simulink model "gm_sampleModel1894_4_sub"  (R2023a)
settings: Solver=VariableStepAuto  StartTime=0.0  StopTime=10.0  RelTol=1e-3
libraries: simulink x3
settings Model: Creator=user1  LastModifiedBy=user1
settings OptimizationCC: BlockReduction=off  ConditionallyExecuteInputs=off
settings DebuggingCC: InheritedTsInSrcMsg=none

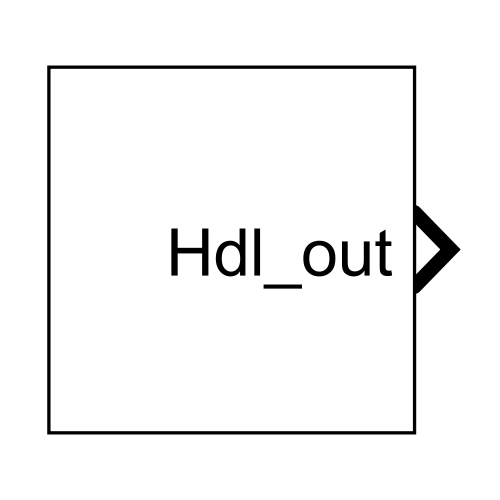
[thumbnail: Simulink's stored preview of the top-level diagram]
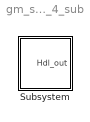
== system gm_sampleModel1894_4_sub ==
  Subsystem : Subsystem

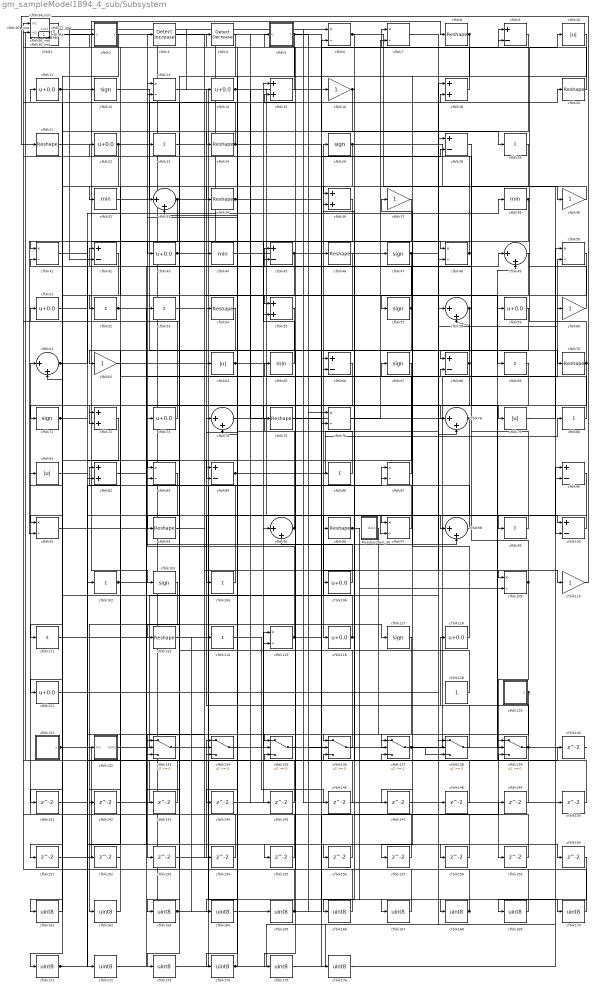
== system gm_sampleModel1894_4_sub/Subsystem ==
  Mysubsystem_30 : Subsystem
  cfblk1 : simulink/Logic and Bit Operations/Detect Increase  vinit=0.0  OutDataTypeStr=uint8
      settings: LibrarySourceBlock=|
      | hdlsllib/Logic and Bit
      | Operations/Detect
      | Increase
  cfblk{10,64,79,81} (4 alike) : Abs  OutDataTypeStr=uint8  SaturateOnIntegerOverflow=off
  cfblk{9,28,42,45,66,68,84,90,100} (9 alike) : Sum  Inputs=+-  OutDataTypeStr=uint8
  cfblk101_inst : Subsystem
  cfblk{23,29,52..53,69,80,86,99,102,104,111,114} (12 alike) : Sum  Inputs=+  OutDataTypeStr=uint8
  cfblk{12,26,47,57,67,71,103,117} (8 alike) : Signum
  cfblk{11,14,22,43,51,59,73,106,116,118,121} (11 alike) : Bias  Bias=0.0  SaturateOnIntegerOverflow=off
  cfblk{6..7,13,41,48,50,76,83,87,91,97,109,115} (13 alike) : Product  Inputs=*/  OutDataTypeStr=uint8  RndMeth=Zero  SaturateOnIntegerOverflow=on
  cfblk{16,37,40,60,62,110} (6 alike) : Gain  OutDataTypeStr=uint8
  cfblk{8,20..21,24,34,46,54,70,75,93,96,113} (12 alike) : Reshape
  cfblk120_inst : Subsystem
  cfblk128 : Constant  OutDataTypeStr=uint8  SampleTime=-1
  cfblk129 : Subsystem  mask(Counter Free-Running){NumBits=double(16), tsamp=double(-1)}
      mask prompts: NumBits "Simulink:masks:NumberOfBits_MP"; tsamp "Simulink:masks:SampleTime_MP"
      mask help: Simulink:masks:CounterFreeRunning_MD
  cfblk131 : Subsystem  mask(Counter Limited){uplimit=double(7), tsamp=double(-1)}
      mask prompts: uplimit "Simulink:masks:UpperLimit_MP"; tsamp "Simulink:masks:SampleTime_MP"
      mask help: Simulink:masks:CounterLimited_MD
      mask init:
      | nbits = double(8);
      | tsamp = double(-1);
      | uplimit = double(7);
  cfblk132 : Subsystem
  cfblk{133..139} (7 alike) : Switch  OutDataTypeStr=uint8  SaturateOnIntegerOverflow=off  InputSameDT=off
  cfblk{140..160} (21 alike) : Delay  SampleTime=1
  cfblk{15,18,36,55,72,82} (6 alike) : Sum  OutDataTypeStr=uint8
  cfblk{161..176} (16 alike) : DataTypeConversion  OutDataTypeStr=uint8  SaturateOnIntegerOverflow=off  RndMeth=Floor
  cfblk2 : Subsystem  mask(Compare To Constant){relop=<=, const=double(3), OutDataTypeStr=uint8, ZeroCross=on}
      mask prompts: relop "Simulink:masks:Operator_MP"; const "Simulink:masks:ConstantValue_MP"; OutDataTypeStr "Simulink:masks:OutputDataType_MP"; ZeroCross "Simulink:masks:EnableZerocrossingDetection_MP"
      mask help: Simulink:masks:CompareToConstant_MD
      mask init:
      | OutDataTypeStr = 'uint8';
      | ZeroCross = 'on';
      | blkName = 'sampleModel1894_4_sub/Subsystem/cfblk2';
      | const = double(3);
      | const_str = '3.0';
      | const_val = double(3);
      | relop = '<=';
      | setValue = 'fixdt(0, 8)';
      | str = '<= 3';
      mask TypeOptions relop: == | ~= | < | <= | >= | >
      mask TypeOptions OutDataTypeStr: Simulink:masks:uint8 | Simulink:masks:boolean
      mask Callback ZeroCross: sl('zeroCrossEnable', gcbh);
      mask Display: disp(str)
  cfblk3 : simulink/Logic and Bit Operations/Detect Increase  vinit=0.0  OutDataTypeStr=uint8
      settings: LibrarySourceBlock=|
      | hdlsllib/Logic and Bit
      | Operations/Detect
      | Increase
  cfblk30_inst : Subsystem
  cfblk{32,39,44,65} (4 alike) : MinMax  OutDataTypeStr=uint8
  cfblk{33,49,58,61,74,78,95,98} (8 alike) : Sum  Inputs=|++  OutDataTypeStr=uint8
  cfblk4 : simulink/Logic and Bit Operations/Detect Decrease  vinit=0.0  OutDataTypeStr=uint8
      settings: LibrarySourceBlock=|
      | hdlsllib/Logic and Bit
      | Operations/Detect
      | Decrease
  cfblk5 : Subsystem  mask(Detect Fall Negative){vinit=double(0), InputProcessing=Elements as channels (sample based), OutDataTypeStr=uint8}
      mask prompts: vinit "Simulink:masks:InitialCondition_MP"; InputProcessing "Simulink:masks:InputProcessing_MP"; OutDataTypeStr "Simulink:masks:OutputDataType_MP"
      mask help: Simulink:masks:DetectFallNegative_MD
      mask init:
      | InputProcessing = 'Elements as channels (sample based)';
      | OutDataTypeStr = 'uint8';
      | vinit = double(0);
      mask TypeOptions InputProcessing: Simulink:masks:ColumnsAsChannelsFrameBased | Simulink:masks:ElementsAsChannelsSampleBased
      mask TypeOptions OutDataTypeStr: Simulink:masks:uint8 | Simulink:masks:boolean
      mask Display: fprintf('U < 0\n&  NOT\nU/z < 0')
  cfblk56_inst : Subsystem
  cfblk77_inst : Subsystem
  cfblk94_inst : Subsystem
  Hdl_out : Outport  OutDataTypeStr=uint8  SampleTime=1
  wires:
  Mysubsystem_30/1(Out1) -> cfblk135/1
  cfblk1/1 -> cfblk8/1, cfblk103/1
  cfblk10/1 -> cfblk173/1
  cfblk100/1 -> cfblk116/1
  cfblk101_inst/1(out1) -> cfblk94_inst/1(in1)
  cfblk102/1 -> cfblk98/2, cfblk156/1
  cfblk103/1 -> cfblk162/1
  cfblk104/1 -> cfblk3/1
  cfblk106/1 -> cfblk95/2
  cfblk109/1 -> cfblk41/2, cfblk159/1
  cfblk11/1 -> cfblk97/1, cfblk48/1, cfblk151/1
  cfblk110/1 -> cfblk21/1
  cfblk111/1 -> cfblk26/1
  cfblk113/1 -> cfblk155/1
  cfblk114/1 -> cfblk146/1
  cfblk115/1 -> cfblk73/1, cfblk10/1
  cfblk116/1 -> cfblk166/1, cfblk11/1
  cfblk117/1 -> cfblk153/1
  cfblk118/1 -> cfblk37/1
  cfblk12/1 -> cfblk68/1
  cfblk120_inst/1(out1) -> cfblk165/1
  cfblk121/1 -> cfblk18/1
  cfblk128/1 -> cfblk53/1
  cfblk129/1(y) -> cfblk137/2, cfblk133/3
  cfblk13/1 -> cfblk168/1
  cfblk131/1(y) -> cfblk139/3, cfblk132/1(In1)
  cfblk132/1(Out1) -> cfblk48/2
  cfblk133/1 -> cfblk87/1
  cfblk134/1 -> cfblk115/2
  cfblk135/1 -> cfblk46/1
  cfblk136/1 -> cfblk14/1
  cfblk137/1 -> cfblk138/3, cfblk50/2
  cfblk138/1 -> cfblk118/1
  cfblk139/1 -> cfblk54/1, cfblk136/3
  cfblk14/1 -> cfblk100/1, cfblk145/1
  cfblk140/1 -> cfblk1/1
  cfblk141/1 -> cfblk172/1
  cfblk142/1 -> cfblk138/1
  cfblk143/1 -> cfblk30_inst/2(in2)
  cfblk144/1 -> cfblk139/1
  cfblk145/1 -> cfblk115/1
  cfblk146/1 -> cfblk101_inst/2(in2)
  cfblk147/1 -> cfblk78/2
  cfblk148/1 -> cfblk36/2
  cfblk149/1 -> cfblk138/2
  cfblk15/1 -> cfblk30_inst/1(in1)
  cfblk150/1 -> cfblk77_inst/2(in2)
  cfblk151/1 -> cfblk6/2
  cfblk152/1 -> cfblk82/1
  cfblk153/1 -> cfblk134/1
  cfblk154/1 -> cfblk42/1
  cfblk155/1 -> cfblk61/1
  cfblk156/1 -> cfblk15/2
  cfblk157/1 -> cfblk134/3
  cfblk158/1 -> cfblk94_inst/2(in2)
  cfblk159/1 -> cfblk45/1
  cfblk16/1 -> cfblk24/1, cfblk106/1
  cfblk160/1 -> cfblk169/1
  cfblk161/1 -> cfblk81/1
  cfblk162/1 -> cfblk2/1(u)
  cfblk163/1 -> cfblk59/1, cfblk114/1
  cfblk164/1 -> cfblk4/1
  cfblk165/1 -> cfblk51/1, cfblk76/1, cfblk149/1
  cfblk166/1 -> cfblk120_inst/1(in1)
  cfblk167/1 -> cfblk120_inst/2(in2)
  cfblk168/1 -> cfblk75/1, cfblk135/3
  cfblk169/1 -> cfblk13/1
  cfblk170/1 -> cfblk13/2
  cfblk171/1 -> cfblk137/3, cfblk87/2, cfblk140/1
  cfblk172/1 -> cfblk49/1
  cfblk173/1 -> cfblk49/2
  cfblk174/1 -> cfblk74/1, cfblk148/1
  cfblk175/1 -> cfblk90/1
  cfblk176/1 -> cfblk90/2
  cfblk18/1 -> cfblk77_inst/1(in1)
  cfblk2/1(y) -> cfblk161/1
  cfblk20/1 -> cfblk9/1
  cfblk21/1 -> cfblk55/2
  cfblk22/1 -> cfblk18/2, cfblk121/1
  cfblk23/1 -> cfblk109/1
  cfblk24/1 -> cfblk66/1, cfblk101_inst/1(in1)
  cfblk26/1 -> cfblk93/1, cfblk113/1, cfblk40/1, cfblk52/1
  cfblk28/1 -> cfblk78/1
  cfblk29/1 -> cfblk133/1
  cfblk3/1 -> cfblk55/1
  cfblk30_inst/1(out1) -> cfblk6/1
  cfblk32/1 -> cfblk20/1
  cfblk33/1 -> cfblk136/2, cfblk91/1
  cfblk34/1 -> cfblk176/1, cfblk167/1
  cfblk36/1 -> cfblk43/1
  cfblk37/1 -> cfblk82/2
  cfblk39/1 -> cfblk91/2, cfblk157/1
  cfblk4/1 -> cfblk163/1
  cfblk40/1 -> cfblk32/1
  cfblk41/1 -> cfblk102/1
  cfblk42/1 -> cfblk61/2
  cfblk43/1 -> cfblk45/2, cfblk69/1
  cfblk44/1 -> cfblk96/1
  cfblk45/1 -> cfblk71/1, cfblk28/2
  cfblk46/1 -> cfblk62/1
  cfblk47/1 -> cfblk136/1, cfblk110/1
  cfblk48/1 -> cfblk56_inst/2(in2), cfblk28/1
  cfblk49/1 -> cfblk171/1
  cfblk5/1(Y) -> cfblk74/2, cfblk34/1, cfblk29/1
  cfblk50/1 -> cfblk147/1
  cfblk51/1 -> cfblk98/1
  cfblk52/1 -> cfblk117/1, cfblk76/2
  cfblk53/1 -> cfblk70/1
  cfblk54/1 -> cfblk83/1
  cfblk55/1 -> cfblk164/1
  cfblk56_inst/1(out1) -> cfblk150/1
  cfblk57/1 -> cfblk72/2, cfblk137/1, cfblk44/1
  cfblk58/1 -> cfblk143/1, cfblk142/1
  cfblk59/1 -> cfblk175/1
  cfblk6/1 -> cfblk36/1, cfblk100/2
  cfblk60/1 -> cfblk7/1
  cfblk61/1 -> cfblk158/1, cfblk39/1
  cfblk62/1 -> cfblk95/1
  cfblk64/1 -> cfblk68/2, cfblk139/2
  cfblk65/1 -> cfblk15/1
  cfblk66/1 -> cfblk72/1
  cfblk67/1 -> cfblk144/1
  cfblk68/1 -> cfblk66/2, cfblk58/2, cfblk152/1
  cfblk69/1 -> cfblk141/1
  cfblk7/1 -> cfblk58/1
  cfblk70/1 -> cfblk9/2, cfblk135/2
  cfblk71/1 -> cfblk84/2, cfblk99/1
  cfblk72/1 -> cfblk111/1
  cfblk73/1 -> cfblk56_inst/1(in1)
  cfblk74/1 -> cfblk79/1
  cfblk75/1 -> cfblk160/1
  cfblk76/1 -> cfblk7/2
  cfblk77_inst/1(out1) -> cfblk47/1, cfblk16/1
  cfblk78/1 -> cfblk97/2, Hdl_out/1, cfblk104/1
  cfblk79/1 -> cfblk50/1
  cfblk8/1 -> cfblk84/1, cfblk57/1
  cfblk80/1 -> cfblk22/1
  cfblk81/1 -> cfblk134/2
  cfblk82/1 -> cfblk65/1
  cfblk83/1 -> cfblk133/2
  cfblk84/1 -> cfblk60/1, cfblk80/1
  cfblk86/1 -> cfblk5/1(U)
  cfblk87/1 -> cfblk67/1
  cfblk9/1 -> cfblk41/1
  cfblk90/1 -> cfblk174/1
  cfblk91/1 -> cfblk64/1
  cfblk93/1 -> cfblk154/1
  cfblk94_inst/1(out1) -> cfblk42/2, cfblk12/1
  cfblk95/1 -> cfblk33/2, cfblk33/1
  cfblk96/1 -> cfblk170/1, cfblk109/2
  cfblk97/1 -> cfblk86/1
  cfblk98/1 -> cfblk83/2
  cfblk99/1 -> cfblk23/1

== system gm_sampleModel1894_4_sub/Subsystem/Mysubsystem_30 ==
  cfblk130 : Subsystem  mask(Counter Free-Running){NumBits=double(16), tsamp=double(-1)}
      mask prompts: NumBits "Simulink:masks:NumberOfBits_MP"; tsamp "Simulink:masks:SampleTime_MP"
      mask help: Simulink:masks:CounterFreeRunning_MD
  cfblk63 : MinMax
  Out1 : Outport  SampleTime=1
  wires:
  cfblk130/1(y) -> cfblk63/1
  cfblk63/1 -> Out1/1

== system gm_sampleModel1894_4_sub/Subsystem/cfblk101_inst ==
  in1 : Inport  OutDataTypeStr=uint8  SampleTime=1
  in2 : Inport  Port=2  OutDataTypeStr=uint8  SampleTime=1
  mul_cfblk101_dotp_mulcomp : Product  Inputs=**  OutDataTypeStr=uint8  SampleTime=1
  out1 : Outport  OutDataTypeStr=uint8  SampleTime=1
  wires:
  in1/1 -> mul_cfblk101_dotp_mulcomp/1
  in2/1 -> mul_cfblk101_dotp_mulcomp/2
  mul_cfblk101_dotp_mulcomp/1 -> out1/1

== system gm_sampleModel1894_4_sub/Subsystem/cfblk120_inst ==
  in1 : Inport  OutDataTypeStr=uint8  SampleTime=1
  in2 : Inport  Port=2  OutDataTypeStr=uint8  SampleTime=1
  mul_cfblk120_dotp_mulcomp : Product  Inputs=**  OutDataTypeStr=uint8  SampleTime=1
  out1 : Outport  OutDataTypeStr=uint8  SampleTime=1
  wires:
  in1/1 -> mul_cfblk120_dotp_mulcomp/1
  in2/1 -> mul_cfblk120_dotp_mulcomp/2
  mul_cfblk120_dotp_mulcomp/1 -> out1/1

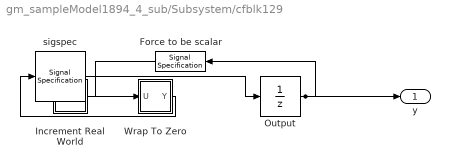
== system gm_sampleModel1894_4_sub/Subsystem/cfblk129 ==
  Force to be scalar : SignalSpecification  DisableCoverage=on  Dimensions=1
  Increment Real World : Subsystem  mask(Real World Value Increment){}
      mask help: Simulink:masks:RealWorldValueIncrement_MD
      mask Display: disp('V++')
  Output : UnitDelay  InitialCondition=0.0  SampleTime=tsamp  HasFrameUpgradeWarning=on
  Wrap To Zero : Subsystem  mask(Wrap To Zero){Threshold=double(65535)}
      mask prompts: Threshold "Simulink:masks:Threshold_MP"
      mask help: Simulink:masks:WrapToZero_MD
  sigspec : SignalSpecification  OutDataTypeStr=uint16  Dimensions=1
  y : Outport  SampleTime=1
  wires:
  Force to be scalar/1 -> Increment Real World/1(u)
  Increment Real World/1(y) -> Wrap To Zero/1(U)
  Output/1 -> Force to be scalar/1, y/1
  Wrap To Zero/1(Y) -> sigspec/1
  sigspec/1 -> Output/1

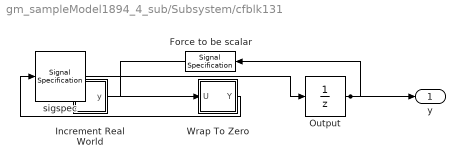
== system gm_sampleModel1894_4_sub/Subsystem/cfblk131 ==
  Force to be scalar : SignalSpecification  DisableCoverage=on  Dimensions=1
  Increment Real World : Subsystem  mask(Real World Value Increment){}
      mask help: Simulink:masks:RealWorldValueIncrement_MD
      mask Display: disp('V++')
  Output : UnitDelay  InitialCondition=0.0  SampleTime=tsamp  HasFrameUpgradeWarning=on
  Wrap To Zero : Subsystem  mask(Wrap To Zero){Threshold=double(7)}
      mask prompts: Threshold "Simulink:masks:Threshold_MP"
      mask help: Simulink:masks:WrapToZero_MD
  sigspec : SignalSpecification  OutDataTypeStr=uint8  Dimensions=1
  y : Outport  SampleTime=1
  wires:
  Force to be scalar/1 -> Increment Real World/1(u)
  Increment Real World/1(y) -> Wrap To Zero/1(U)
  Output/1 -> Force to be scalar/1, y/1
  Wrap To Zero/1(Y) -> sigspec/1
  sigspec/1 -> Output/1

== system gm_sampleModel1894_4_sub/Subsystem/cfblk132 ==
  In1 : Inport  OutDataTypeStr=uint8  PortDimensions=1  SampleTime=1
  Out1 : Outport  SampleTime=1
  wires:
  In1/1 -> Out1/1

== system gm_sampleModel1894_4_sub/Subsystem/cfblk2 ==
  u : Inport  OutDataTypeStr=uint8  SampleTime=1
  Compare : RelationalOperator  Operator=<=  OutDataTypeStr=fixdt(0, 8)
  Constant : Constant  DisableCoverage=on  Value=const  OutDataTypeStr=Inherit: Inherit via back propagation  SampleTime=-1
  y : Outport  SampleTime=1
  wires:
  u/1 -> Compare/1
  Compare/1 -> y/1
  Constant/1 -> Compare/2

== system gm_sampleModel1894_4_sub/Subsystem/cfblk30_inst ==
  in1 : Inport  OutDataTypeStr=uint8  SampleTime=1
  in2 : Inport  Port=2  OutDataTypeStr=uint8  SampleTime=1
  mul_cfblk30_dotp_mulcomp : Product  Inputs=**  OutDataTypeStr=uint8  SampleTime=1
  out1 : Outport  OutDataTypeStr=uint8  SampleTime=1
  wires:
  in1/1 -> mul_cfblk30_dotp_mulcomp/1
  in2/1 -> mul_cfblk30_dotp_mulcomp/2
  mul_cfblk30_dotp_mulcomp/1 -> out1/1

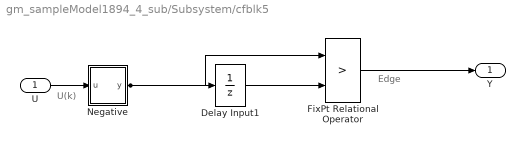
== system gm_sampleModel1894_4_sub/Subsystem/cfblk5 ==
  note: U(k)
  note: Edge
  U : Inport  OutDataTypeStr=uint8  SampleTime=1
  Delay Input1 : UnitDelay  Description=Store in Global RAM  DisableCoverage=on  InitialCondition=vinit  SampleTime=-1  HasFrameUpgradeWarning=on
  FixPt Relational Operator : RelationalOperator  Operator=>  OutDataTypeStr=fixdt(0, 8)  ZeroCross=off  InputSameDT=off
  Negative : Subsystem  mask(Compare To Zero){relop=<, OutDataTypeStr=boolean, ZeroCross=off}
      mask prompts: relop "Simulink:masks:Operator_MP"; OutDataTypeStr "Simulink:masks:OutputDataType_MP"; ZeroCross "Simulink:masks:EnableZerocrossingDetection_MP"
      mask help: Simulink:masks:CompareToZero_MD
      mask init:
      | OutDataTypeStr = 'boolean';
      | ZeroCross = 'off';
      | blkName = 'sampleModel1894_4_sub/Subsystem/cfblk5/Negative';
      | relop = '<';
      | setValue = 'boolean';
      mask TypeOptions relop: == | ~= | < | <= | >= | >
      mask TypeOptions OutDataTypeStr: Simulink:masks:uint8 | Simulink:masks:boolean
      mask Callback ZeroCross: sl('zeroCrossEnable', gcbh);
      mask Display: disp([relop,' 0'])
  Y : Outport  SampleTime=1
  wires:
  U/1 -> Negative/1(u)
  Delay Input1/1 -> FixPt Relational Operator/2
  FixPt Relational Operator/1 -> Y/1
  Negative/1(y) -> FixPt Relational Operator/1, Delay Input1/1

== system gm_sampleModel1894_4_sub/Subsystem/cfblk56_inst ==
  in1 : Inport  OutDataTypeStr=uint8  SampleTime=1
  in2 : Inport  Port=2  OutDataTypeStr=uint8  SampleTime=1
  mul_cfblk56_dotp_mulcomp : Product  Inputs=**  OutDataTypeStr=uint8  SampleTime=1
  out1 : Outport  OutDataTypeStr=uint8  SampleTime=1
  wires:
  in1/1 -> mul_cfblk56_dotp_mulcomp/1
  in2/1 -> mul_cfblk56_dotp_mulcomp/2
  mul_cfblk56_dotp_mulcomp/1 -> out1/1

== system gm_sampleModel1894_4_sub/Subsystem/cfblk77_inst ==
  in1 : Inport  OutDataTypeStr=uint8  SampleTime=1
  in2 : Inport  Port=2  OutDataTypeStr=uint8  SampleTime=1
  mul_cfblk77_dotp_mulcomp : Product  Inputs=**  OutDataTypeStr=uint8  SampleTime=1
  out1 : Outport  OutDataTypeStr=uint8  SampleTime=1
  wires:
  in1/1 -> mul_cfblk77_dotp_mulcomp/1
  in2/1 -> mul_cfblk77_dotp_mulcomp/2
  mul_cfblk77_dotp_mulcomp/1 -> out1/1

== system gm_sampleModel1894_4_sub/Subsystem/cfblk94_inst ==
  in1 : Inport  OutDataTypeStr=uint8  SampleTime=1
  in2 : Inport  Port=2  OutDataTypeStr=uint8  SampleTime=1
  mul_cfblk94_dotp_mulcomp : Product  Inputs=**  OutDataTypeStr=uint8  SampleTime=1
  out1 : Outport  OutDataTypeStr=uint8  SampleTime=1
  wires:
  in1/1 -> mul_cfblk94_dotp_mulcomp/1
  in2/1 -> mul_cfblk94_dotp_mulcomp/2
  mul_cfblk94_dotp_mulcomp/1 -> out1/1

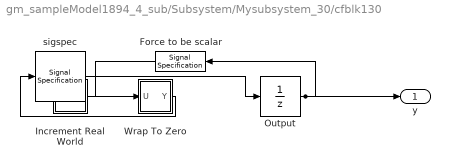
== system gm_sampleModel1894_4_sub/Subsystem/Mysubsystem_30/cfblk130 ==
  Force to be scalar : SignalSpecification  DisableCoverage=on  Dimensions=1
  Increment Real World : Subsystem  mask(Real World Value Increment){}
      mask help: Simulink:masks:RealWorldValueIncrement_MD
      mask Display: disp('V++')
  Output : UnitDelay  InitialCondition=0.0  SampleTime=tsamp  HasFrameUpgradeWarning=on
  Wrap To Zero : Subsystem  mask(Wrap To Zero){Threshold=double(65535)}
      mask prompts: Threshold "Simulink:masks:Threshold_MP"
      mask help: Simulink:masks:WrapToZero_MD
  sigspec : SignalSpecification  OutDataTypeStr=uint16  Dimensions=1
  y : Outport  SampleTime=1
  wires:
  Force to be scalar/1 -> Increment Real World/1(u)
  Increment Real World/1(y) -> Wrap To Zero/1(U)
  Output/1 -> Force to be scalar/1, y/1
  Wrap To Zero/1(Y) -> sigspec/1
  sigspec/1 -> Output/1

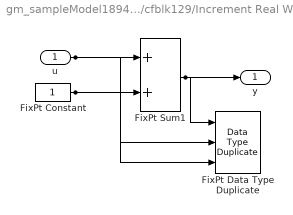
== system gm_sampleModel1894_4_sub/Subsystem/cfblk129/Increment Real World ==
  u : Inport  OutDataTypeStr=uint16  SampleTime=1
  FixPt Constant : Constant  DisableCoverage=on  OutDataTypeStr=Inherit: Inherit via back propagation  SampleTime=-1
  FixPt Data Type Duplicate : DataTypeDuplicate  DisableCoverage=on  NumInputPorts=3
  FixPt Sum1 : Sum  InputSameDT=on  OutDataTypeStr=Inherit: Inherit via back propagation  LockScale=on
  y : Outport  SampleTime=1
  wires:
  u/1 -> FixPt Sum1/1, FixPt Data Type Duplicate/2
  FixPt Constant/1 -> FixPt Sum1/2, FixPt Data Type Duplicate/3
  FixPt Sum1/1 -> FixPt Data Type Duplicate/1, y/1

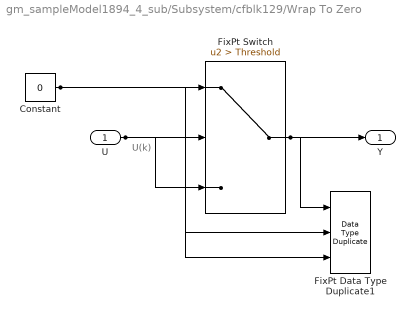
== system gm_sampleModel1894_4_sub/Subsystem/cfblk129/Wrap To Zero ==
  note: U(k)
  U : Inport  OutDataTypeStr=uint16  SampleTime=1
  Constant : Constant  DisableCoverage=on  Value=0  OutDataTypeStr=Inherit: Inherit via back propagation  SampleTime=-1
  FixPt Data Type Duplicate1 : DataTypeDuplicate  DisableCoverage=on  NumInputPorts=3
  FixPt Switch : Switch  Criteria=u2 > Threshold  Threshold=Threshold  OutDataTypeStr=Inherit: Inherit via back propagation  ZeroCross=off  SaturateOnIntegerOverflow=off  InputSameDT=off
  Y : Outport  SampleTime=1
  wires:
  U/1 -> FixPt Switch/3, FixPt Switch/2, FixPt Data Type Duplicate1/2
  Constant/1 -> FixPt Switch/1, FixPt Data Type Duplicate1/3
  FixPt Switch/1 -> FixPt Data Type Duplicate1/1, Y/1

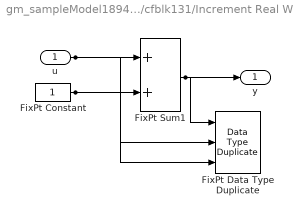
== system gm_sampleModel1894_4_sub/Subsystem/cfblk131/Increment Real World ==
  u : Inport  OutDataTypeStr=uint8  SampleTime=1
  FixPt Constant : Constant  DisableCoverage=on  OutDataTypeStr=Inherit: Inherit via back propagation  SampleTime=-1
  FixPt Data Type Duplicate : DataTypeDuplicate  DisableCoverage=on  NumInputPorts=3
  FixPt Sum1 : Sum  InputSameDT=on  OutDataTypeStr=Inherit: Inherit via back propagation  LockScale=on
  y : Outport  SampleTime=1
  wires:
  u/1 -> FixPt Sum1/1, FixPt Data Type Duplicate/2
  FixPt Constant/1 -> FixPt Sum1/2, FixPt Data Type Duplicate/3
  FixPt Sum1/1 -> FixPt Data Type Duplicate/1, y/1

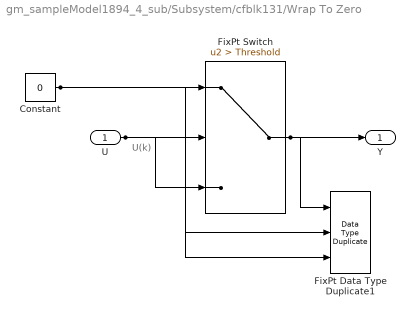
== system gm_sampleModel1894_4_sub/Subsystem/cfblk131/Wrap To Zero ==
  note: U(k)
  U : Inport  OutDataTypeStr=uint8  SampleTime=1
  Constant : Constant  DisableCoverage=on  Value=0  OutDataTypeStr=Inherit: Inherit via back propagation  SampleTime=-1
  FixPt Data Type Duplicate1 : DataTypeDuplicate  DisableCoverage=on  NumInputPorts=3
  FixPt Switch : Switch  Criteria=u2 > Threshold  Threshold=Threshold  OutDataTypeStr=Inherit: Inherit via back propagation  ZeroCross=off  SaturateOnIntegerOverflow=off  InputSameDT=off
  Y : Outport  SampleTime=1
  wires:
  U/1 -> FixPt Switch/3, FixPt Switch/2, FixPt Data Type Duplicate1/2
  Constant/1 -> FixPt Switch/1, FixPt Data Type Duplicate1/3
  FixPt Switch/1 -> FixPt Data Type Duplicate1/1, Y/1

== system gm_sampleModel1894_4_sub/Subsystem/cfblk5/Negative ==
  u : Inport  OutDataTypeStr=uint8  SampleTime=1
  Compare : RelationalOperator  Operator=<  OutDataTypeStr=boolean  ZeroCross=off
  Constant : Constant  DisableCoverage=on  Value=0  OutDataTypeStr=Inherit: Inherit via back propagation  SampleTime=-1  PreserveConstantTs=on
  y : Outport  SampleTime=1
  wires:
  u/1 -> Compare/1
  Compare/1 -> y/1
  Constant/1 -> Compare/2

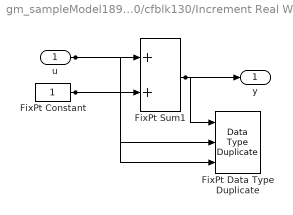
== system gm_sampleModel1894_4_sub/Subsystem/Mysubsystem_30/cfblk130/Increment Real World ==
  u : Inport  OutDataTypeStr=uint16  SampleTime=1
  FixPt Constant : Constant  DisableCoverage=on  OutDataTypeStr=Inherit: Inherit via back propagation  SampleTime=-1
  FixPt Data Type Duplicate : DataTypeDuplicate  DisableCoverage=on  NumInputPorts=3
  FixPt Sum1 : Sum  InputSameDT=on  OutDataTypeStr=Inherit: Inherit via back propagation  LockScale=on
  y : Outport  SampleTime=1
  wires:
  u/1 -> FixPt Sum1/1, FixPt Data Type Duplicate/2
  FixPt Constant/1 -> FixPt Sum1/2, FixPt Data Type Duplicate/3
  FixPt Sum1/1 -> FixPt Data Type Duplicate/1, y/1

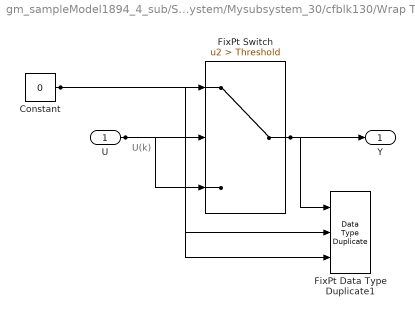
== system gm_sampleModel1894_4_sub/Subsystem/Mysubsystem_30/cfblk130/Wrap To Zero ==
  note: U(k)
  U : Inport  OutDataTypeStr=uint16  SampleTime=1
  Constant : Constant  DisableCoverage=on  Value=0  OutDataTypeStr=Inherit: Inherit via back propagation  SampleTime=-1
  FixPt Data Type Duplicate1 : DataTypeDuplicate  DisableCoverage=on  NumInputPorts=3
  FixPt Switch : Switch  Criteria=u2 > Threshold  Threshold=Threshold  OutDataTypeStr=Inherit: Inherit via back propagation  ZeroCross=off  SaturateOnIntegerOverflow=off  InputSameDT=off
  Y : Outport  SampleTime=1
  wires:
  U/1 -> FixPt Switch/3, FixPt Switch/2, FixPt Data Type Duplicate1/2
  Constant/1 -> FixPt Switch/1, FixPt Data Type Duplicate1/3
  FixPt Switch/1 -> FixPt Data Type Duplicate1/1, Y/1
